simulink model "simpleMotor"  (R2018b)
settings: Solver=FixedStepAuto  StartTime=0.0  StopTime=20.0  RelTol=1e-3  EnableMultiTasking=on
libraries: arduinolib x2, dspstat3 x2
settings Model: SimulationMode=external  ExtModeTrigDuration=2  Creator=bill  LastModifiedBy=bill
settings OptimizationCC: EnhancedBackFolding=on  PassReuseOutputArgsAs=Individual arguments  MaxStackSize=64  OptimizeBlockOrder=speed  DifferentSizesBufferReuse=on  OptimizationCustomize=off
settings DebuggingCC: ParameterTunabilityLossMsg=error
settings HardwareCC: ProdBitPerInt=16  ProdBitPerPointer=16  ProdBitPerSizeT=16  ProdBitPerPtrDiffT=16  ProdLargestAtomicFloat=None  ProdWordSize=8  ProdHWDeviceType=Atmel->AVR  UseEmbeddedCoderFeatures=off  UseSimulinkCoderFeatures=off
settings SFSimCC: MATLABDynamicMemAlloc=off
settings RTWCC: SystemTargetFile=ert.tlc  HardwareBoard=Arduino Uno  TemplateMakefile=ert_default_tmf  GenerateReport=on  Toolchain=Arduino AVR  BuildConfiguration=Faster Runs  IncludeHyperlinkInReport=on  LaunchReport=on  GenerateTraceInfo=on  GenerateTraceReport=on  GenerateTraceReportSl=on  GenerateTraceReportSf=on  GenerateTraceReportEml=on
settings CodeAppCC: ForceParamTrailComments=on  IgnoreCustomStorageClasses=off  OperatorAnnotations=on  SimulinkDataObjDesc=on  SFDataObjDesc=on  InsertBlockDesc=on
settings ERTTargetCC: SupportContinuousTime=on  SupportNonInlinedSFcns=on  SupportVariableSizeSignals=on

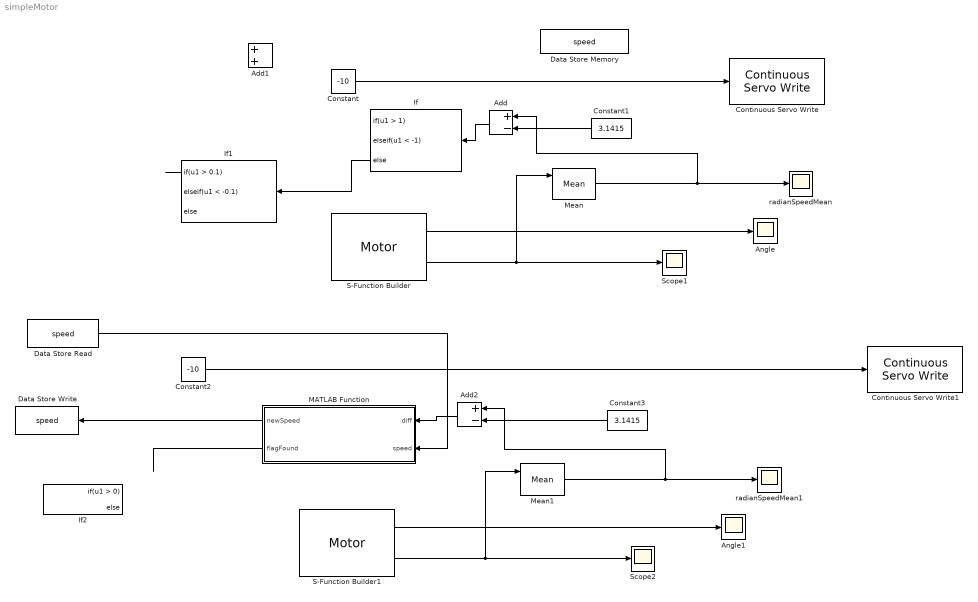
== system simpleMotor ==
  Add : Sum  Inputs=+-
  Add1 : Sum
  Add2 : Sum  Inputs=+-
  Angle : Scope
  Angle1 : Scope
  Constant : Constant  Value=-10
  Constant1 : Constant  Value=3.1415
  Constant2 : Constant  Value=-10
  Constant3 : Constant  Value=3.1415
  Continuous Servo Write : arduinolib/Continuous Servo Write  pinNumber=7  ServoIndex=0  blockPlatform=ARDUINO
      settings: SourceProductName=Simulink Support Package for Arduino Hardware  SourceProductBaseCode=ARDUINO
  Continuous Servo Write1 : arduinolib/Continuous Servo Write  pinNumber=7  ServoIndex=0  blockPlatform=ARDUINO
      settings: SourceProductName=Simulink Support Package for Arduino Hardware  SourceProductBaseCode=ARDUINO
  Data Store Memory : DataStoreMemory  DataStoreName=speed  ReadBeforeWriteMsg=warning  WriteAfterWriteMsg=warning  WriteAfterReadMsg=warning  ShowAdditionalParam=off
  Data Store Read : DataStoreRead  DataStoreName=speed
  Data Store Write : DataStoreWrite  DataStoreName=speed
  If : If  IfExpression=u1 > 1  ElseIfExpressions=u1 < -1
  If1 : If  IfExpression=u1 > 0.1  ElseIfExpressions=u1 < -0.1
  If2 : If
  MATLAB Function : MATLAB Function  TreatAsAtomicUnit=on
  Mean : dspstat3/Mean  run=on  InputProcessing=Columns as channels (frame based)  reset_popup=Rising edge  directionMode=Each column  dimension=1  roiEnable=off  roiType=Rectangles  roiPortion=Entire ROI  roiOutput=Individual statistics for each ROI  roiFlag=off  roundingMode=Floor  overflowMode=off  outputDataTypeStr=Inherit: Same as accumulator  outputMin=[]  outputMax=[]  outputLastDataTypeStr=Inherit: Same as accumulator
  Mean1 : dspstat3/Mean  run=on  InputProcessing=Columns as channels (frame based)  reset_popup=Rising edge  directionMode=Each column  dimension=1  roiEnable=off  roiType=Rectangles  roiPortion=Entire ROI  roiOutput=Individual statistics for each ROI  roiFlag=off  roundingMode=Floor  overflowMode=off  outputDataTypeStr=Inherit: Same as accumulator  outputMin=[]  outputMax=[]  outputLastDataTypeStr=Inherit: Same as accumulator
  S-Function Builder : S-Function  InitFcn=try, set_param(gcb,'FunctionName','Motor'), end  FunctionName=Motor  SFunctionModules=Motor_wrapper  SFunctionDeploymentMode=off  EnableBusSupport=off  mask(S-Function Builder){}
      mask help: Simulink:masks:SFunctionBuilder_MD
      mask init:
      | val = [[.9  0.75 0.75 1 1 .9 .9 1]',[1 1 0.75 0.75 .9 .9 1 .9]'];try , sys = get_param(gcb,'SfunBuilderFcnName');if isempty(sys), sys = get_param(gcb,'FunctionName'); end,catch, sys = get_param(gcb,'FunctionName'); end
      settings: CopyFcn=set_param(gcbh,'LinkStatus','none')  PreSaveFcn=try, set_param(gcb,'FunctionName','Motor'), end  OpenFcn=sfunctionwizard(gcbh)
      mask Display: plot(val(:,1),val(:,2)),disp(sys), port_label('output',1,'posRad'), port_label('output',2,'deriv')
  S-Function Builder1 : S-Function  InitFcn=try, set_param(gcb,'FunctionName','Motor'), end  FunctionName=Motor  SFunctionModules=Motor_wrapper  SFunctionDeploymentMode=off  EnableBusSupport=off  mask(S-Function Builder){}
      mask help: Simulink:masks:SFunctionBuilder_MD
      mask init: same as simpleMotor/S-Function Builder
      settings: CopyFcn=set_param(gcbh,'LinkStatus','none')  PreSaveFcn=try, set_param(gcb,'FunctionName','Motor'), end  OpenFcn=sfunctionwizard(gcbh)
      mask Display: plot(val(:,1),val(:,2)),disp(sys), port_label('output',1,'posRad'), port_label('output',2,'deriv')
  Scope1 : Scope
  Scope2 : Scope
  radianSpeedMean : Scope
  radianSpeedMean1 : Scope
  wires:
  S-Function Builder/1 -> Angle/1
  S-Function Builder/2 -> Mean/1, Scope1/1
  Constant/1 -> Continuous Servo Write/1
  Mean/1 -> Add/1, radianSpeedMean/1
  Constant1/1 -> Add/2
  Add/1 -> If/1
  If/3 -> If1/1
  If1/1 -> ?
  Add2/1 -> MATLAB Function/1(diff)
  Mean1/1 -> Add2/1, radianSpeedMean1/1
  Constant2/1 -> Continuous Servo Write1/1
  S-Function Builder1/2 -> Mean1/1, Scope2/1
  Constant3/1 -> Add2/2
  S-Function Builder1/1 -> Angle1/1
  Data Store Read/1 -> MATLAB Function/2(speed)
  MATLAB Function/1(newSpeed) -> Data Store Write/1
  MATLAB Function/2(flagFound) -> ?

== matlab function simpleMotor/MATLAB Function ==
  data: diff input; newSpeed output; speed input; flagFound output
function [newSpeed,flagFound] = updateSpeed(diff,speed)
if(diff > 1)
    newSpeed = speed + 1;
    flagFound = false;
elseif(diff < -1)
    newSpeed = speed - 1;
    flagFound = false;
else
    if(diff > 0.1)
        newSpeed = speed + 0.1;
        flagFound = false;
    elseif(diff < -0.1)
        newSpeed = speed - 0.1;
        flagFound = false;
    else
        flagFound = true;
        newSpeed = speed;
        disp("speed found");
        disp(newSpeed);
    end
end
end
